simulink model "en_broadcast"  (R2018a)
settings: Solver=VariableStepAuto  StartTime=0.0  StopTime=0.1  RelTol=1e-3
settings Model: Creator=BEAR  LastModifiedBy=BEAR

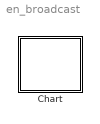
== system en_broadcast ==
  Chart : Stateflow chart  TreatAsAtomicUnit=on

== stateflow chart en_broadcast/Chart ==
  state A
    en: E;f("enA_done")
  state B
    en: f("enB")
  state C
    en: f("enC")
  (default) -> A
  A -> B : E
  B -> C
  data: s function_input
  events: E local FUNCTION_CALL_EVENT
  function f(s):
    | function f(s)
    |   fprintf(s+"\n");
